simulink library "SLoWCBlock"  (R2018b)
settings: Solver=VariableStepAuto  StartTime=0.0  StopTime=10.0  RelTol=1e-3
settings Model: Creator=RA24876  LastModifiedBy=RA24876
settings SFSimCC: SimUseLocalCustomCode=off
settings RTWCC: RTWUseLocalCustomCode=off
settings CodeAppCC: StateflowObjectComments=on

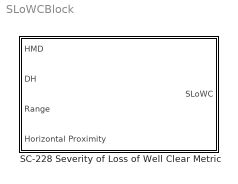
== system SLoWCBlock ==
  SC-228 Severity of Loss of Well Clear Metric : Subsystem  mask(SC-228 Severity of Loss of Well Clear Metric){DMOD=4000, altDiffThreshold=450}
      mask prompts: altDiffThreshold "Altitude Difference Threshold:"
      mask help:
      | Computes the Severity of Loss of Well Clear Metric (SLoWC).  Can be used with the SeverityOfLoWC wrapper class.
      |
      | Takes the following input signals:
      |
      |    HMD - current predicted horizontal miss distance
      |    DH - absolute value of the current vertical separation
      |    Range - current horizontal range
      |    Horizontal Proximity - horizontal extent of the Hazard Zone
      |
      | Returns the maximum value of SLoWC.  Values range from 0 (best) to 1 (worst).

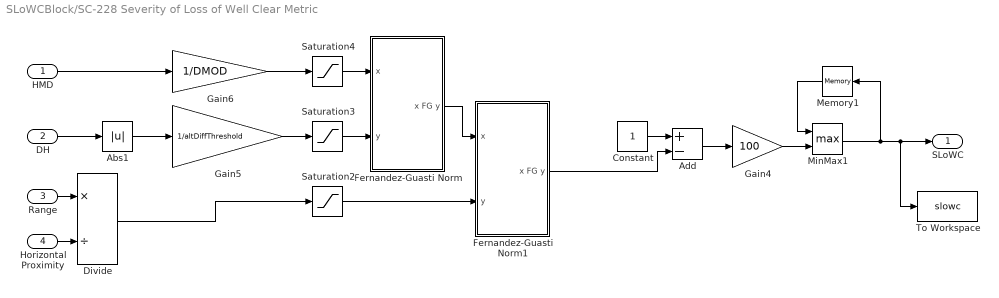
== system SLoWCBlock/SC-228 Severity of Loss of Well Clear Metric ==
  HMD : Inport
  DH : Inport  Port=2
  Range : Inport  Port=3
  Horizontal Proximity : Inport  Port=4
  Abs1 : Abs
  Add : Sum  Inputs=+-
  Constant : Constant
  Divide : Product  Inputs=*/
  Fernandez-Guasti Norm : Subsystem
  Fernandez-Guasti Norm1 : Subsystem
  Gain4 : Gain  Gain=100
  Gain5 : Gain  Gain=1/altDiffThreshold
  Gain6 : Gain  Gain=1/DMOD
  Memory1 : Memory
  MinMax1 : MinMax  Function=max  Inputs=2
  Saturation2 : Saturate  UpperLimit=1  LowerLimit=0  LinearizeAsGain=off
  Saturation3 : Saturate  UpperLimit=1  LowerLimit=0  LinearizeAsGain=off
  Saturation4 : Saturate  UpperLimit=1  LowerLimit=0  LinearizeAsGain=off
  To Workspace : ToWorkspace  VariableName=slowc  SampleTime=-1
      settings: MaxDataPoints=1
  SLoWC : Outport
  wires:
  Divide/1 -> Saturation2/1
  Memory1/1 -> MinMax1/1
  MinMax1/1 -> Memory1/1, To Workspace/1, SLoWC/1
  Saturation4/1 -> Fernandez-Guasti Norm/1(x)
  Add/1 -> Gain4/1
  Constant/1 -> Add/1
  Saturation2/1 -> Fernandez-Guasti Norm1/2(y)
  Fernandez-Guasti Norm/1(x FG y) -> Fernandez-Guasti Norm1/1(x)
  DH/1 -> Abs1/1
  Gain4/1 -> MinMax1/2
  Abs1/1 -> Gain5/1
  Saturation3/1 -> Fernandez-Guasti Norm/2(y)
  Gain5/1 -> Saturation3/1
  HMD/1 -> Gain6/1
  Gain6/1 -> Saturation4/1
  Range/1 -> Divide/1
  Horizontal Proximity/1 -> Divide/2
  Fernandez-Guasti Norm1/1(x FG y) -> Add/2

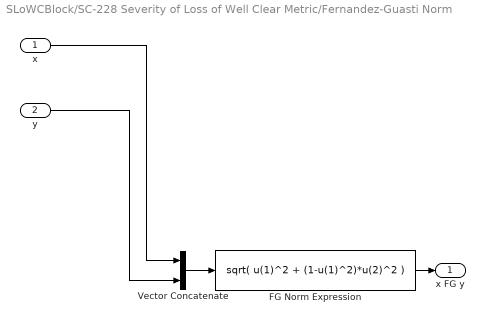
== system SLoWCBlock/SC-228 Severity of Loss of Well Clear Metric/Fernandez-Guasti Norm ==
  x : Inport
  y : Inport  Port=2
  FG Norm Expression : Fcn  Expr=sqrt( u(1)^2 + (1-u(1)^2)*u(2)^2 )
  Vector Concatenate : Concatenate
  x FG y : Outport
  wires:
  y/1 -> Vector Concatenate/2
  x/1 -> Vector Concatenate/1
  FG Norm Expression/1 -> x FG y/1
  Vector Concatenate/1 -> FG Norm Expression/1

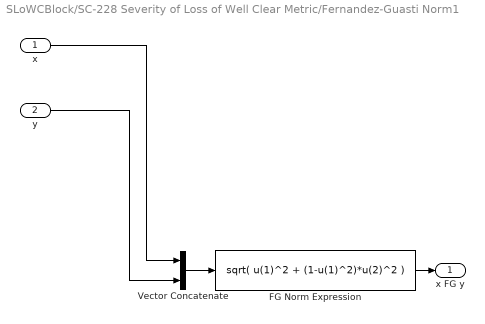
== system SLoWCBlock/SC-228 Severity of Loss of Well Clear Metric/Fernandez-Guasti Norm1 ==
  x : Inport
  y : Inport  Port=2
  FG Norm Expression : Fcn  Expr=sqrt( u(1)^2 + (1-u(1)^2)*u(2)^2 )
  Vector Concatenate : Concatenate
  x FG y : Outport
  wires:
  y/1 -> Vector Concatenate/2
  x/1 -> Vector Concatenate/1
  FG Norm Expression/1 -> x FG y/1
  Vector Concatenate/1 -> FG Norm Expression/1
